simulink model "example02"  (R2022a)
settings: Solver=VariableStepAuto  StartTime=0.0  StopTime=10.0  RelTol=1e-3
settings Model: Creator=mluser  LastModifiedBy=cunis
settings ModelReferenceCC: EnableRefExpFcnMdlSchedulingChecks=off
settings RTWCC: Description=Generic Real-Time Target

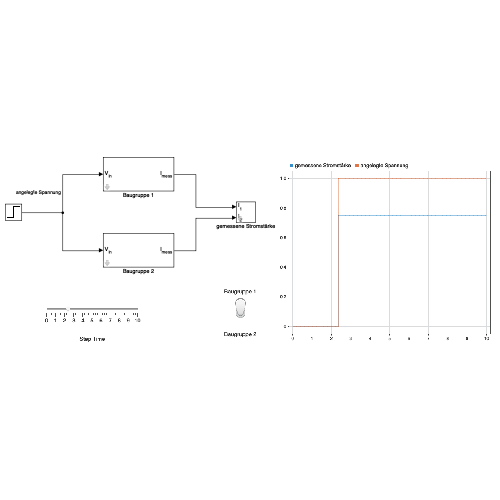
[thumbnail: Simulink's stored preview of the top-level diagram]
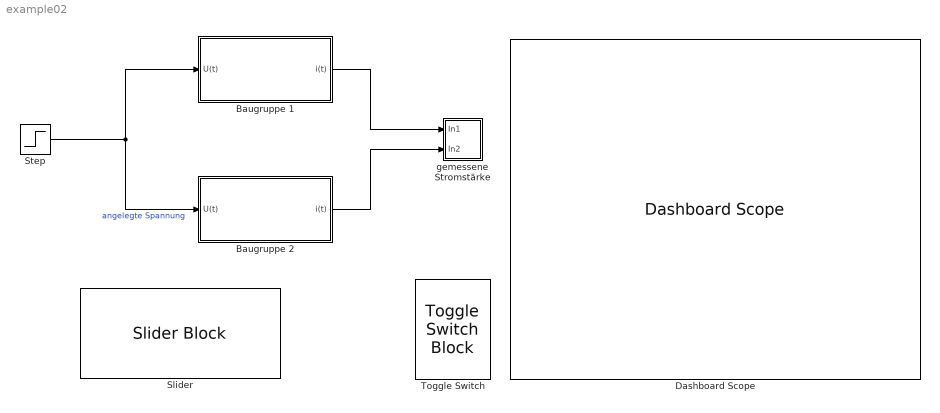
== system example02 ==
  Baugruppe 1 : Subsystem
      mask Display:
      | port_label('input', 1, 'V_{in}', 'interpreter', 'tex');
      | port_label('output', 1, 'I_{mess}', 'interpreter', 'tex');
  Baugruppe 2 : Subsystem
      mask Display:
      | port_label('input', 1, 'V_{in}', 'interpreter', 'tex');
      | port_label('output', 1, 'I_{mess}', 'interpreter', 'tex');
  Dashboard Scope : DashboardScope
  Slider : SliderBlock  LabelPosition=Bottom  ScaleMax=10
  Step : Step  Time=2.339396284829721  SampleTime=0
  Toggle Switch : ToggleSwitchBlock  LabelPosition=Hide
      settings: Values={{'Baugruppe 2', 'Baugruppe 1'}, [0 1]}
  gemessene Stromstärke : Subsystem
      mask Display:
      | port_label('input', 1, 'I_1', 'interpreter', 'tex');
      | port_label('input', 2, 'I_2', 'interpreter', 'tex');
  wires:
  Step/1 -> Baugruppe 2/1(U(t)), Baugruppe 1/1(U(t))  "angelegte Spannung"
  Baugruppe 1/1(i(t)) -> gemessene Stromstärke/1(In1)
  Baugruppe 2/1(i(t)) -> gemessene Stromstärke/2(In2)

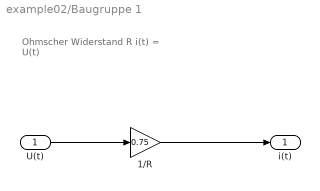
== system example02/Baugruppe 1 ==
  note: Ohmscher Widerstand
      | R i(t) = U(t)
  U(t) : Inport
  1/R : Gain  Gain=0.75
  i(t) : Outport
  wires:
  U(t)/1 -> 1/R/1
  1/R/1 -> i(t)/1

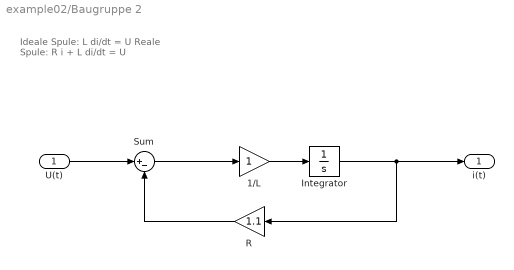
== system example02/Baugruppe 2 ==
  note: Ideale Spule:
      | L di/dt = U
      |
      | Reale Spule:
      | R i + L di/dt = U
  U(t) : Inport
  1/L : Gain
  Integrator : Integrator
  R : Gain  Gain=1.1
  Sum : Sum  Inputs=|+-
  i(t) : Outport
  wires:
  U(t)/1 -> Sum/1
  1/L/1 -> Integrator/1
  Integrator/1 -> R/1, i(t)/1
  Sum/1 -> 1/L/1
  R/1 -> Sum/2

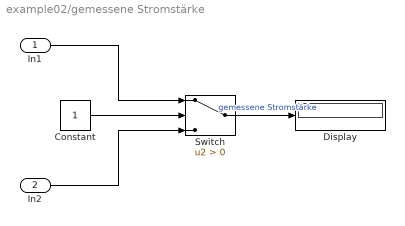
== system example02/gemessene Stromstärke ==
  In1 : Inport
  In2 : Inport  Port=2
  Constant : Constant
  Display : Display
  Switch : Switch  Criteria=u2 > Threshold  SaturateOnIntegerOverflow=off  InputSameDT=off
  wires:
  In1/1 -> Switch/1
  In2/1 -> Switch/3
  Switch/1 -> Display/1  "gemessene Stromstärke"
  Constant/1 -> Switch/2
